simulink model "GhendyanoTrifasico"  (R2021b)
settings: Solver=ode45  StartTime=0.0  StopTime=0.1  RelTol=1e-3  EnableMultiTasking=on
values from neighbouring files (symbols this model uses):
  C_matrix = [7.86602198725e-09  -2.45195546694e-09  -1.42580481937e-09; -2.45195546694e-09  8.37188965904e-09  -2.45195546694e-09; -1.42580481937e-09  -2.45195546694e-09  7.86602198725e-09]    [trif2awg.mat]
  L_matrix = [0.00242085814129  0.00130892171515  0.00117029227904; 0.00130892171515  0.00242085814129  0.00130892171515; 0.00117029227904  0.00130892171515  0.00242085814129]    [trif2awg.mat]
  R_matrix = [1.15895092862  0.0568724513894  0.0568719145431; 0.0568724513894  1.15895092862  0.0568724513894; 0.0568719145431  0.0568724513894  1.15895092862]    [trif2awg.mat]
  RaF = n    [Ghendyano.m]
undefined symbols (not defined in the file or in its folder): D11, Delta
libraries: spsThreePhaseVIMeasurementLib x2, spsCurrentMeasurementLib x1, spsDistributedParametersLineLib x1, spsGroundLib x1, spsSeriesRLCBranchLib x1, spsThreePhaseTransformerTwoWindingsLib x1, spsThreePhaseSourceLib x1, spspowerguiLib x1
settings Model: Creator=laris  LastModifiedBy=LeonardoFelipe
settings SolverCC: AlgebraicLoopSolver=TrustRegion
settings DataIOCC: LimitDataPoints=on  SaveFormat=Array  ReturnWorkspaceOutputs=off
settings OptimizationCC: LifeSpan=inf
settings DebuggingCC: SFUnexpectedBacktrackingDiag=warning  SFNoUnconditionalDefaultTransitionDiag=warning  SFExecutionAtInitializationDiag=none  SFMachineParentedDataDiag=warning  ArithmeticOperatorsInVariantConditions=warning
settings HardwareCC: ProdBitPerPointer=32  ProdBitPerSizeT=32  ProdBitPerPtrDiffT=32  ProdLargestAtomicFloat=None  ProdIntDivRoundTo=Undefined  ProdEndianess=Unspecified  ProdWordSize=32  ProdHWDeviceType=32-bit Generic
settings ModelReferenceCC: PropagateSignalLabelsOutOfModel=off
settings SFSimCC: SimUseLocalCustomCode=off  CustomCodeUndefinedFunction=UseInterfaceOnly
settings RTWCC: RTWUseLocalCustomCode=off
settings CodeAppCC: StateflowObjectComments=on
settings GRTTargetCC: TargetLangStandard=C89/C90 (ANSI)
settings ConfigComp: CovMetricSettings=dw  CovSaveCumulativeToWorkspaceVar=on  CovSaveSingleToWorkspaceVar=on  CovExternalEMLEnable=off
settings SimscapeCC: SimscapeNormalizeSystem=off

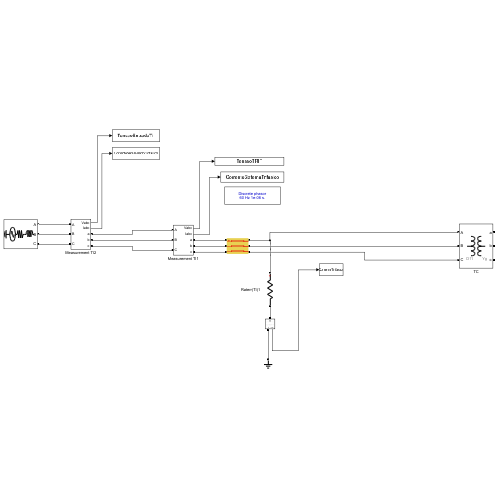
[thumbnail: Simulink's stored preview of the top-level diagram]
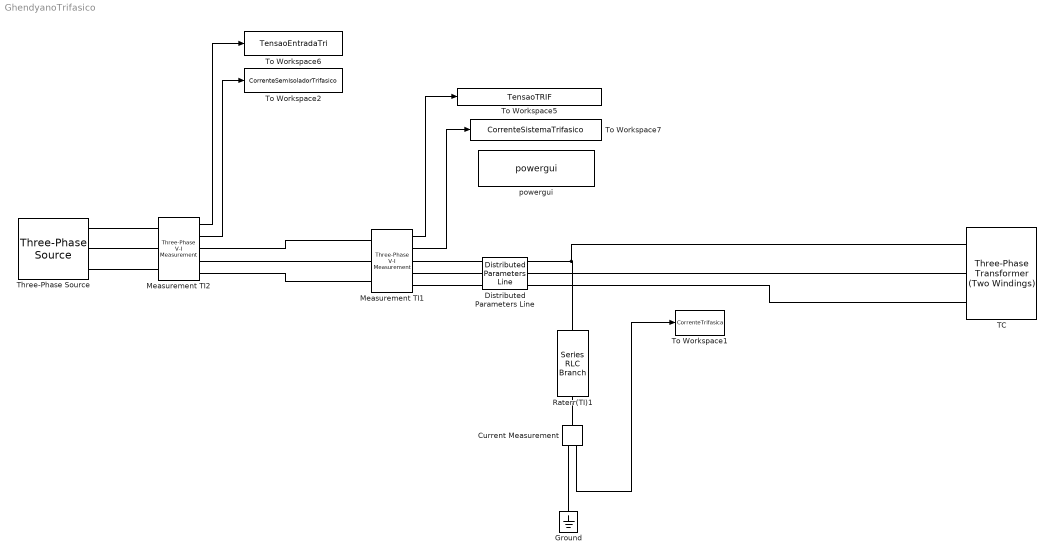
== system GhendyanoTrifasico ==
  Current Measurement : spsCurrentMeasurementLib/Current Measurement  PhasorSimulation=on  OutputType=Complex  PSBequivalent=0
  Distributed Parameters Line : spsDistributedParametersLineLib/Distributed Parameters Line  Phases=3  Length=m1  Frequency=60  Resistance=R_matrix  Inductance=L_matrix  Capacitance=C_matrix  x1=[312.003612765819 7946.31993784959 7917.87492875433;376.991118430775 376.991118430775 376.991118430775;-2.25366827622477 -0.610674096373514 -2.17006488400207]  x2=[5790.26472652774 4515.66543430078 7801.51850100117;376.991118430775 376.991118430775 376.991118430775;-2.9076807520499 -0.836153902038433 -1.90128547800075]  x3=[39.7957392225538 28.0542235271658 36.665971442261;376.991118430775 376.991118430775 376.991118430775;2.37452474915323 2.34131253519076 -1.39214669901029]  x4=[37.2242665529678 57.5702937396462 27.3089490462134;376.991118430775 376.991118430775 376.991118430775;-0.880502041868955 -0.765534212423557 -3.09303374438256]  x5=0.000260355177502627  V1=ones(3,3)  V2=ones(3,3)  I1=ones(3,3)  I2=ones(3,3)  nHarmo=1  Measurements=None  Decoupling=off  VsMag0=0  VrMag0=0  VsAngle0=0  VrAngle0=0  IsMag0=0  IrMag0=0  IsAngle0=0  IrAngle0=0
      settings: SourceProductBaseCode=PS
  Ground : spsGroundLib/Ground  LConnTagsString=a
  Measurement TI1 : spsThreePhaseVIMeasurementLib/Three-Phase V-I Measurement  VoltageMeasurement=phase-to-phase  SetLabelV=off  LabelV=Vabc  Vpu=off  VpuLL=off  CurrentMeasurement=yes  SetLabelI=off  LabelI=Iabc  Ipu=off  Pbase=100e6  Vbase=500e3  OutputType=Complex  PhasorSimulation=on  PSBequivalent=0
  Measurement TI2 : spsThreePhaseVIMeasurementLib/Three-Phase V-I Measurement  VoltageMeasurement=phase-to-phase  SetLabelV=off  LabelV=Vabc  Vpu=off  VpuLL=off  CurrentMeasurement=yes  SetLabelI=off  LabelI=Iabc  Ipu=off  Pbase=100e6  Vbase=500e3  OutputType=Magnitude  PhasorSimulation=on  PSBequivalent=0
  Raterr(TI)1 : spsSeriesRLCBranchLib/Series RLC Branch  LConnTagsString=__new0  RConnTagsString=__new0  BranchType=R  Resistance=RaF  Inductance=0  SetiL0=off  InitialCurrent=0  Capacitance=1e-6  Setx0=off  InitialVoltage=0  Measurements=None
  TC : spsThreePhaseTransformerTwoWindingsLib/Three-Phase Transformer (Two Windings)  Winding1Connection=Delta (D11)  Winding2Connection=Yg  CoreType=Three single-phase transformers  SetSaturation=off  Hysteresis=off  DataFile='hysteresis'  SetInitialFlux=off  Measurements=None  UNITS=pu  NominalPower=[300e3 , 60]  Winding1=[13800 0.0048118 0.018511]  Winding2=[380 0.0048119 0.018511]  Rm=5.801193266567229e+02*1000  Lm=8.409977380031759e+02*1000  L0=0.50001  Saturation=[0 0;0.0012545 0.01913;0.52272 0.024231]  InitialFluxes=[0.66025 -0.66025 0.57767]  BreakLoop=off  DiscreteSolver=Trapezoidal iterative  DataType=off  TransfoNumber=1
  Three-Phase Source : spsThreePhaseSourceLib/Three-Phase Source  InternalConnection=Yg  VoltagePhases=off  Voltage=13.8e3/sqrt(3)  PhaseAngle=0  Voltage_phases=[25e3 25e3 25e3]/sqrt(3)  PhaseAngles_phases=[0 -120 +120]  Frequency=60  NonIdealSource=on  SpecifyImpedance=on  Resistance=0.8929  Inductance=16.58e-3  ShortCircuitLevel=120e6  BaseVoltage=13.8e3  XRratio=7  BusType=swing  Pref=10e3  Qref=0  Prefabc=[10e3, 10e3, 10e3]  Qrefabc=[0, 0, 0]  Qmin=-inf  Qmax=inf
  To Workspace1 : ToWorkspace  VariableName=CorrenteTrifasica  SampleTime=-1
      settings: MaxDataPoints=1
  To Workspace2 : ToWorkspace  VariableName=CorrenteSemIsoladorTrifasico  SampleTime=-1
      settings: MaxDataPoints=1
  To Workspace5 : ToWorkspace  VariableName=TensaoTRIF  SampleTime=-1
      settings: MaxDataPoints=1
  To Workspace6 : ToWorkspace  VariableName=TensaoEntradaTri  SampleTime=-1
      settings: MaxDataPoints=1
  To Workspace7 : ToWorkspace  VariableName=CorrenteSistemaTrifasico  SampleTime=-1
      settings: MaxDataPoints=1
  powergui : spspowerguiLib/powergui  Priority=1  SimulationMode=Discrete phasor  SampleTime=1e-6  frequency=60  Iterations=50  frequencyindice=60  Pbase=100e6  ErrMax=1e-4  UnitsV=kV  UnitsW=MW  buscounter=0  FunctionMessages=off  echomessages=off  EnableUseOfTLC=off  CurrentSourceSwitches=off  DisableSnubberDevices=off  DisableRonSwitches=off  DisableVfSwitches=off  DisplayEquations=off  AutomaticDiscreteSolvers=off  SolverType=Tustin/Backward Euler (TBE)  Interpol=off  ExternalGateDelay=off  methode=off  Ts=100  x0status=blocks  SPID=on  SwTol=0  HookPort=off  NonlinearTolerance=1e-4  nMaxIteration=100  ContinueOnMaxIteration=off  RestoreLinks=warning  ResistiveCurrentMeasurement=off  Frange=[0:2:500]  Ylog=off  Xlog=on  ShowGrid=off  save=off  variable=ZData  structure=0  ZoomFFT=off  StartTime=0.0  cycles=1  DisplayStyle=1  fundamental=60  FreqAxis=off  MaxFrequency=1000  frequencyindicesteady=1  RmsSteady=1  display=off
  wires:
  Measurement TI1/1 -> To Workspace5/1
  Measurement TI2/1 -> To Workspace6/1
  Measurement TI2/2 -> To Workspace2/1
  Current Measurement/1 -> To Workspace1/1
  Measurement TI1/2 -> To Workspace7/1
  connections:
  Measurement TI2/RConn2 -- Measurement TI1/LConn2
  Measurement TI2/RConn3 -- Measurement TI1/LConn3
  Three-Phase Source/RConn3 -- Measurement TI2/LConn3
  Three-Phase Source/RConn2 -- Measurement TI2/LConn2
  Three-Phase Source/RConn1 -- Measurement TI2/LConn1
  Measurement TI1/LConn1 -- Measurement TI2/RConn1
  Measurement TI1/RConn1 -- Distributed Parameters Line/LConn1
  Raterr(TI)1/LConn1 -- TC/LConn1 -- Distributed Parameters Line/RConn1
  Current Measurement/LConn1 -- Raterr(TI)1/RConn1
  Current Measurement/RConn1 -- Ground/LConn1
  Measurement TI1/RConn2 -- Distributed Parameters Line/LConn2
  Distributed Parameters Line/LConn3 -- Measurement TI1/RConn3
  TC/LConn2 -- Distributed Parameters Line/RConn2
  Distributed Parameters Line/RConn3 -- TC/LConn3
